simulink model "TrafficLight_SFD"  (R2016a)
settings: Solver=FixedStepDiscrete  StartTime=0.0  StopTime=7  FixedStep=0.1  RelTol=1e-3
settings Model: Creator=DELL  LastModifiedBy=DELL
settings SolverCC: AutoInsertRateTranBlk=on
settings DataIOCC: LimitDataPoints=on
settings OptimizationCC: DefaultParameterBehavior=Inlined  UseDivisionForNetSlopeComputation=on  UseFloatMulNetSlope=on  InlineInvariantSignals=on  PassReuseOutputArgsAs=Individual arguments  ZeroExternalMemoryAtStartup=off  ZeroInternalMemoryAtStartup=off  NoFixptDivByZeroProtection=on  EfficientFloat2IntCast=on  OptimizeModelRefInitCode=on  LifeSpan=1
settings DebuggingCC: AllowSymbolicDim=off
settings RTWCC: SystemTargetFile=ert.tlc  TemplateMakefile=ert_default_tmf  GenerateReport=on  IncludeHyperlinkInReport=on  LaunchReport=on  GenerateTraceInfo=on  GenerateTraceReport=on  GenerateTraceReportSl=on  GenerateTraceReportSf=on  GenerateTraceReportEml=on  GenerateCodeMetricsReport=on
settings CodeAppCC: ForceParamTrailComments=on  IgnoreCustomStorageClasses=off  OperatorAnnotations=on  SimulinkDataObjDesc=on  SFDataObjDesc=on  MATLABFcnDesc=on  CustomSymbolStrGlobalVar=rt$N$M  CustomSymbolStrType=$N$M  CustomSymbolStrFcn=$N$M$F  CustomSymbolStrMacro=$N$M  InsertBlockDesc=on  MATLABSourceComments=on
settings ERTTargetCC: GenerateSampleERTMain=on  IncludeMdlTerminateFcn=off  CombineSignalStateStructs=on  SupportAbsoluteTime=off  SupportComplex=off  SupportNonInlinedSFcns=on  InlinedParameterPlacement=NonHierarchical  ERTCustomFileTemplate=example_file_process.tlc  ERTFilePackagingFormat=CompactWithDataFile
settings ConfigComp: CovModelRefEnable=Off  CovSFcnEnable=off

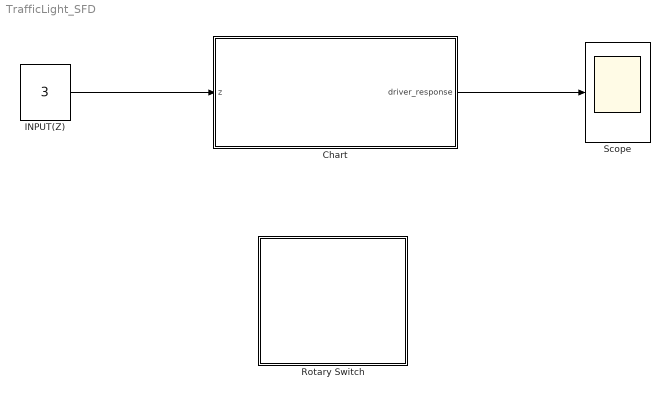
== system TrafficLight_SFD ==
  Chart : Stateflow chart  TreatAsAtomicUnit=on
  INPUT(Z) : Constant  Value=3
  Rotary Switch : Subsystem  DialogController=hmiCreateDDGDialog  IsWebBlock=on  mask(MWDashboardBlock){webBlockId=e83749ed-597f-46d3-a0ed-202abfa5dcf0, webBlockType=discreteknob, ShowInLibBrowser=on, ShowInitialText=on, HMISrcModelName=TrafficLight_SFD}
      mask prompts: webBlockId "WebBlock Id"; webBlockType "WebBlock Type"; HMISrcModelName "Source Model"
      mask Help: helpview([docroot '/mapfiles/simulink.map'], 'hmi_rotary_switch')
      mask Display:
      | model = bdroot(gcb);
      | if strcmp(get_param(model,'BlockDiagramType'), 'library')
      |     image([(matlabroot) '/toolbox/simulink/hmi/icons/DiscreteKnob.png']);
      | end
  Scope : Scope
  wires:
  Chart/1(driver_response) -> Scope/1
  INPUT(Z)/1 -> Chart/1(z)

== system TrafficLight_SFD/Rotary Switch ==

== stateflow chart TrafficLight_SFD/Chart ==
  state START
  state YELLOW
    entry: driver_response=0
  state RED
    entry: driver_response=1
  state GREEN
    entry: driver_response=0
  state CAR_BEGINS_TO_MOVE
    entry: driver_response=0.5;
  state CAR_BEGINS_TO_STOP
    entry: driver_response=0.5
  state CAR_MOVES
    entry: driver_response=1;
  state CAR_STOPS_COMPLETELY
    entry: driver_response=0;
  (default) -> START
  START -> GREEN [order 1] : [z==1]
  START -> RED [order 3] : [z==3]
  START -> YELLOW [order 2] : [z==2]
  RED -> CAR_BEGINS_TO_STOP : [after(1,sec)]
  GREEN -> CAR_BEGINS_TO_MOVE : [after(1,sec)]
  CAR_BEGINS_TO_MOVE -> CAR_MOVES : [after(1,sec)]
  CAR_BEGINS_TO_STOP -> CAR_STOPS_COMPLETELY : [after(1,sec)]
  data: z input; driver_response output
